simulink model "L0203"  (Simulink 9.1)
settings: Solver=VariableStepAuto  StartTime=0.0  StopTime=20  RelTol=1e-3
libraries: simulink x2
settings Model: Creator=Asus  LastModifiedBy=Asus
settings DataIOCC: SaveFormat=Dataset
settings OptimizationCC: LifeSpan=auto
settings DebuggingCC: UnderspecifiedInitializationDetection=Simplified  MergeDetectMultiDrivingBlocksExec=error  SFUnexpectedBacktrackingDiag=error  SFNoUnconditionalDefaultTransitionDiag=error  SFExecutionAtInitializationDiag=warning
settings HardwareCC: ProdBitPerPointer=64  ProdBitPerSizeT=64  ProdBitPerPtrDiffT=64  ProdLargestAtomicFloat=Float  ProdIntDivRoundTo=Zero  ProdEndianess=LittleEndian  ProdWordSize=64  ProdHWDeviceType=Intel->x86-64 (Windows64)
settings ModelReferenceCC: PropagateSignalLabelsOutOfModel=on
settings CodeAppCC: StateflowObjectComments=off
settings GRTTargetCC: TargetLangStandard=C99 (ISO)  CombineOutputUpdateFcns=on  GRTInterface=off
settings ConfigComp: CovMetricSettings=dwe  CovHtmlReporting=off  CovSaveCumulativeToWorkspaceVar=off  CovSaveSingleToWorkspaceVar=off  CovExternalEMLEnable=on

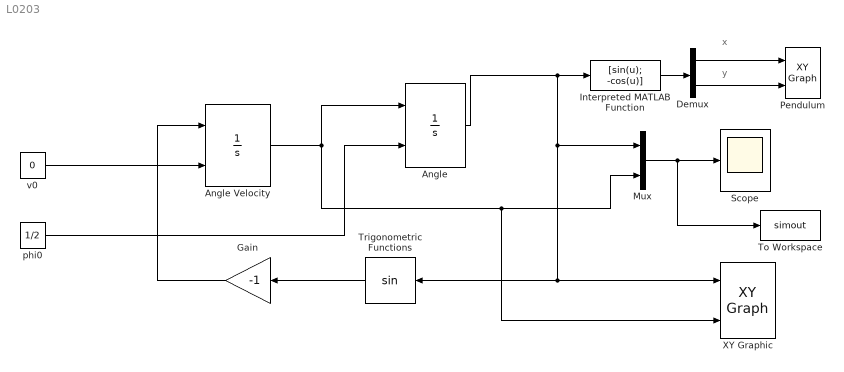
== system L0203 ==
  note: x
  note: y
  Angle : Integrator  InitialConditionSource=external
  Angle Velocity : Integrator  InitialConditionSource=external
  Demux : Demux  Outputs=2
  Gain : Gain  Gain=-1
  Interpreted MATLAB Function : MATLABFcn  MATLABFcn=[sin(u); -cos(u)]  OutputDimensions=2
  Mux : Mux  Inputs=2
  "Pendulum " : simulink/Sinks/XY Graph  xmin=-1  xmax=1  ymin=-1  ymax=1  st=-1
  Scope : Scope
  To Workspace : ToWorkspace  VariableName=simout  SaveFormat=Timeseries  SampleTime=-1
  Trigonometric Functions : Trigonometry
  "XY Graphic " : simulink/Sinks/XY Graph  xmin=-1  xmax=1  ymin=-1  ymax=1  st=-1
  "phi0 " : Constant  Value=1/2
  "v0 " : Constant  Value=0
  wires:
  Angle Velocity/1 -> "XY Graphic "/2, Mux/2, Angle/1
  Gain/1 -> Angle Velocity/1
  Mux/1 -> To Workspace/1, Scope/1
  Trigonometric Functions/1 -> Gain/1
  Angle/1 -> Trigonometric Functions/1, "XY Graphic "/1, Mux/1, Interpreted MATLAB Function/1
  "phi0 "/1 -> Angle/2
  "v0 "/1 -> Angle Velocity/2
  Interpreted MATLAB Function/1 -> Demux/1
  Demux/2 -> "Pendulum "/2
  Demux/1 -> "Pendulum "/1
